simulink model "PD3_DCS_810698349"  (R2021b)
settings: Solver=VariableStepAuto  StartTime=0.0  StopTime=0.1  RelTol=1e-3
undefined symbols (not defined in the file): Ad, C, C_d, G, g, G_d, H, K, Kc, L, L_d, L_p, M, N, R, Ts, wd, y0, y00
settings Model: Creator=SinaK  LastModifiedBy=SinaK

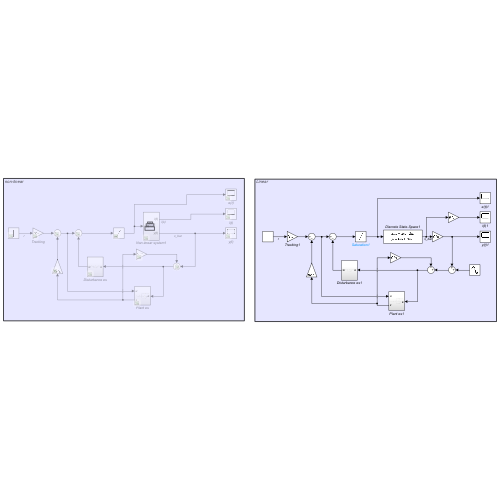
[thumbnail: Simulink's stored preview of the top-level diagram]
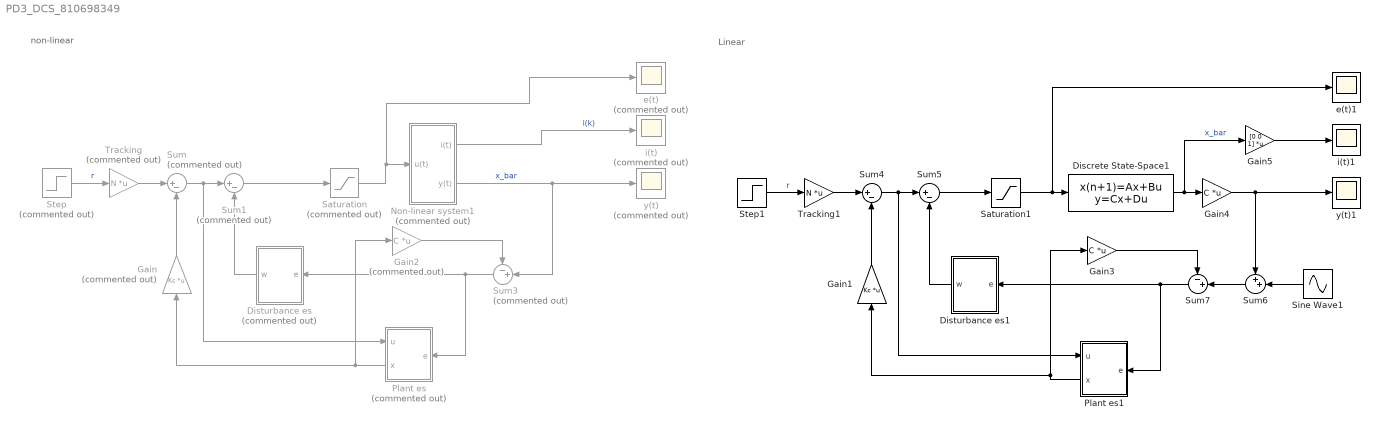
== system PD3_DCS_810698349 ==
  note: Linear
  note: non-linear
  Discrete State-Space1 : DiscreteStateSpace  A=G  B=H  C=eye(3)  D=[0;0;0]  InitialCondition=[y00 0 0]  SampleTime=Ts
  Disturbance es : Subsystem  Commented=on
      settings: PortSchema="{\"entries\":[{\"content\":{\"sides\":[{\"content\":{\"connectorIds\":[\"Out1\"]},\"type\":\"ConnectorPlacement.EquallySpacedRectSide\",\"uuid\":\"7dd2fe88-ba23-450d-b62f-d7570c7d4a9a\"},{\"content\":{\"connectorIds\":[\"In1\"],\"side\":\"RIGHT\"},\"type\":\"ConnectorPlacement.EquallySpacedRectSide\",\"uuid\":\"0a4220da-270b-4baa-869a-0910f399fc2e\"},{\"content\":{\"connectorIds\":[],\"side\":\"TOP\"},\"type\":\"ConnectorPlacement.EquallySpacedRectSide\",\"uuid\":\"bb1cd4e3-8afb-4066-b34f-6b8e4218f629\"}]},\"type\":\"ConnectorPlacement.EquallySpacedConnector\",\"uuid\":\"247f8fe5-253d-4e7a-bc0a-d05e429903fb\"}],\"packageUris\":[\"http://schema.mathworks.com/mf0/Connector/R2020b\"],\"version\":\"1.0\"}"
  Disturbance es1 : Subsystem
      settings: PortSchema="{\"entries\":[{\"content\":{\"sides\":[{\"content\":{\"connectorIds\":[\"Out1\"]},\"type\":\"ConnectorPlacement.EquallySpacedRectSide\",\"uuid\":\"7dd2fe88-ba23-450d-b62f-d7570c7d4a9a\"},{\"content\":{\"connectorIds\":[\"In1\"],\"side\":\"RIGHT\"},\"type\":\"ConnectorPlacement.EquallySpacedRectSide\",\"uuid\":\"0a4220da-270b-4baa-869a-0910f399fc2e\"},{\"content\":{\"connectorIds\":[],\"side\":\"TOP\"},\"type\":\"ConnectorPlacement.EquallySpacedRectSide\",\"uuid\":\"bb1cd4e3-8afb-4066-b34f-6b8e4218f629\"}]},\"type\":\"ConnectorPlacement.EquallySpacedConnector\",\"uuid\":\"247f8fe5-253d-4e7a-bc0a-d05e429903fb\"}],\"packageUris\":[\"http://schema.mathworks.com/mf0/Connector/R2020b\"],\"version\":\"1.0\"}"
  Gain : Gain  Commented=on  Gain=Kc  Multiplication=Matrix(K*u)
  Gain1 : Gain  Gain=Kc  Multiplication=Matrix(K*u)
  Gain2 : Gain  Commented=on  Gain=C  Multiplication=Matrix(K*u)
  Gain3 : Gain  Gain=C  Multiplication=Matrix(K*u)
  Gain4 : Gain  Gain=C  Multiplication=Matrix(K*u)
  Gain5 : Gain  Gain=[0 0 1]  Multiplication=Matrix(K*u)
  Non-linear system1 : Subsystem  Commented=on
  Plant es : Subsystem  Commented=on
      settings: PortSchema="{\"entries\":[{\"content\":{\"sides\":[{\"content\":{\"connectorIds\":[\"In1\",\"Out1\"]},\"type\":\"ConnectorPlacement.EquallySpacedRectSide\",\"uuid\":\"314f560e-5b7f-4e5c-b02d-8249f7ba5ae3\"},{\"content\":{\"connectorIds\":[\"In2\"],\"side\":\"RIGHT\"},\"type\":\"ConnectorPlacement.EquallySpacedRectSide\",\"uuid\":\"7b9ed6a2-80f4-4af4-bb8e-da5172d833a4\"},{\"content\":{\"connectorIds\":[],\"side\":\"TOP\"},\"type\":\"ConnectorPlacement.EquallySpacedRectSide\",\"uuid\":\"b6b0ea98-fd65-4c0a-95e2-ca3e605f4d55\"}]},\"type\":\"ConnectorPlacement.EquallySpacedConnector\",\"uuid\":\"1548adc4-d2fc-42af-9b44-933c6ce86982\"}],\"packageUris\":[\"http://schema.mathworks.com/mf0/Connector/R2020b\"],\"version\":\"1.0\"}"
  Plant es1 : Subsystem
      settings: PortSchema="{\"entries\":[{\"content\":{\"sides\":[{\"content\":{\"connectorIds\":[\"In1\",\"Out1\"]},\"type\":\"ConnectorPlacement.EquallySpacedRectSide\",\"uuid\":\"314f560e-5b7f-4e5c-b02d-8249f7ba5ae3\"},{\"content\":{\"connectorIds\":[\"In2\"],\"side\":\"RIGHT\"},\"type\":\"ConnectorPlacement.EquallySpacedRectSide\",\"uuid\":\"7b9ed6a2-80f4-4af4-bb8e-da5172d833a4\"},{\"content\":{\"connectorIds\":[],\"side\":\"TOP\"},\"type\":\"ConnectorPlacement.EquallySpacedRectSide\",\"uuid\":\"b6b0ea98-fd65-4c0a-95e2-ca3e605f4d55\"}]},\"type\":\"ConnectorPlacement.EquallySpacedConnector\",\"uuid\":\"1548adc4-d2fc-42af-9b44-933c6ce86982\"}],\"packageUris\":[\"http://schema.mathworks.com/mf0/Connector/R2020b\"],\"version\":\"1.0\"}"
  Saturation : Saturate  Commented=on  UpperLimit=12  LowerLimit=0
  Saturation1 : Saturate  UpperLimit=12  LowerLimit=0
  Sine Wave1 : Sin  Amplitude=Ad/M  Frequency=wd  SampleTime=Ts
  Step : Step  Commented=on  Time=0  After=y0  SampleTime=Ts
  Step1 : Step  Time=0  After=y0  SampleTime=Ts
  Sum : Sum  Commented=on  Inputs=|+-
  Sum1 : Sum  Commented=on  Inputs=|+-
  Sum3 : Sum  Commented=on  Inputs=-+|
  Sum4 : Sum  Inputs=|+-
  Sum5 : Sum  Inputs=|+-
  Sum6 : Sum  Inputs=++|
  Sum7 : Sum  Inputs=-+|
  Tracking : Gain  Commented=on  Gain=N  Multiplication=Matrix(K*u)
  Tracking1 : Gain  Gain=N  Multiplication=Matrix(K*u)
  e(t) : Scope  Commented=on
  e(t)1 : Scope
  i(t) : Scope  Commented=on
  i(t)1 : Scope
  y(t) : Scope  Commented=on
  y(t)1 : Scope
  wires:
  Step/1 -> Tracking/1  "r"
  Tracking/1 -> Sum/1
  Sum/1 -> Plant es/1(u), Sum1/1
  Non-linear system1/2(y(t)) -> y(t)/1, Sum3/2  "x_bar"
  Gain/1 -> Sum/2
  Plant es/1(x) -> Gain2/1, Gain/1
  Disturbance es/1(w) -> Sum1/2
  Sum3/1 -> Disturbance es/1(e), Plant es/2(e)
  Gain2/1 -> Sum3/1
  Saturation/1 -> e(t)/1, Non-linear system1/1(u(t))
  Sum1/1 -> Saturation/1
  Non-linear system1/1(i(t)) -> i(t)/1  "i(k)"
  Sum4/1 -> Plant es1/1(u), Sum5/1
  Step1/1 -> Tracking1/1  "r"
  Gain3/1 -> Sum7/1
  Gain1/1 -> Sum4/2
  Tracking1/1 -> Sum4/1
  Sum7/1 -> Disturbance es1/1(e), Plant es1/2(e)
  Plant es1/1(x) -> Gain3/1, Gain1/1
  Disturbance es1/1(w) -> Sum5/2
  Saturation1/1 -> e(t)1/1, Discrete State-Space1/1
  Sum5/1 -> Saturation1/1
  Discrete State-Space1/1 -> Gain5/1, Gain4/1  "x_bar"
  Gain4/1 -> Sum6/1, y(t)1/1
  Gain5/1 -> i(t)1/1
  Sum6/1 -> Sum7/2
  Sine Wave1/1 -> Sum6/2

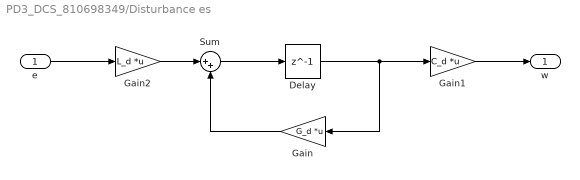
== system PD3_DCS_810698349/Disturbance es ==
  e : Inport
  Delay : Delay  DelayLength=1  SampleTime=Ts
  Gain : Gain  Gain=G_d  Multiplication=Matrix(K*u)
  Gain1 : Gain  Gain=C_d  Multiplication=Matrix(K*u)
  Gain2 : Gain  Gain=L_d  Multiplication=Matrix(K*u)
  Sum : Sum  Inputs=|++
  w : Outport
  wires:
  Sum/1 -> Delay/1
  Gain/1 -> Sum/2
  Delay/1 -> Gain1/1, Gain/1
  Gain1/1 -> w/1
  Gain2/1 -> Sum/1
  e/1 -> Gain2/1

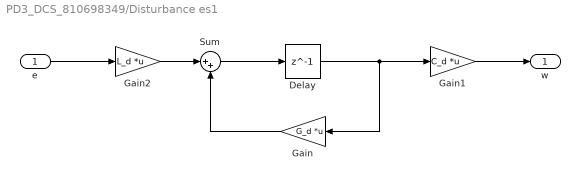
== system PD3_DCS_810698349/Disturbance es1 ==
  e : Inport
  Delay : Delay  DelayLength=1  SampleTime=Ts
  Gain : Gain  Gain=G_d  Multiplication=Matrix(K*u)
  Gain1 : Gain  Gain=C_d  Multiplication=Matrix(K*u)
  Gain2 : Gain  Gain=L_d  Multiplication=Matrix(K*u)
  Sum : Sum  Inputs=|++
  w : Outport
  wires:
  Sum/1 -> Delay/1
  Gain/1 -> Sum/2
  Delay/1 -> Gain1/1, Gain/1
  Gain1/1 -> w/1
  Gain2/1 -> Sum/1
  e/1 -> Gain2/1

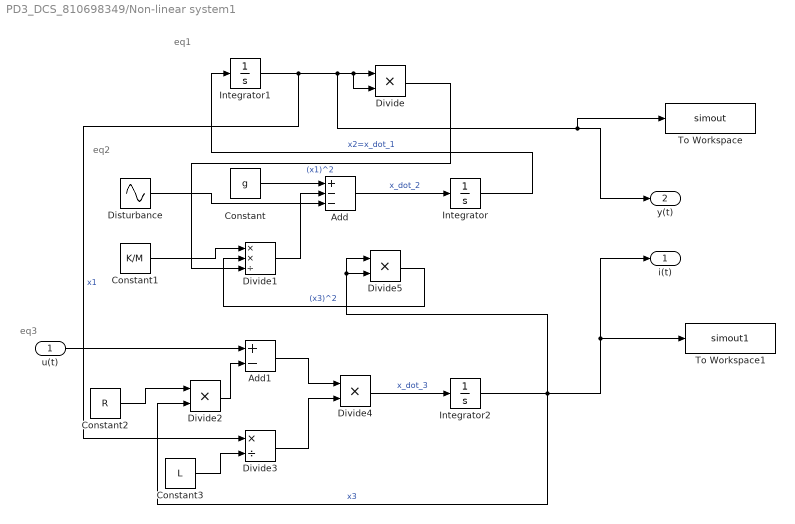
== system PD3_DCS_810698349/Non-linear system1 ==
  note: eq1
  note: eq2
  note: eq3
  u(t) : Inport
  Add : Sum  Inputs=+--
  Add1 : Sum  Inputs=+-
  Constant : Constant  Value=g  SampleTime=Ts
  Constant1 : Constant  Value=K/M  SampleTime=Ts
  Constant2 : Constant  Value=R  SampleTime=Ts
  Constant3 : Constant  Value=L  SampleTime=Ts
  Disturbance : Sin  Amplitude=Ad/M  Frequency=wd  SampleTime=Ts
  Divide{,2,4..5} (4 alike) : Product  Inputs=**
  Divide1 : Product  Inputs=**/
  Divide3 : Product  Inputs=*/
  Integrator : Integrator
  Integrator1 : Integrator  InitialCondition=y00
  Integrator2 : Integrator
  To Workspace : ToWorkspace  VariableName=simout  SaveFormat=Timeseries  SampleTime=-1
      settings: Decimation=3
  To Workspace1 : ToWorkspace  VariableName=simout1  SaveFormat=Timeseries  SampleTime=-1
      settings: Decimation=3
  i(t) : Outport
  y(t) : Outport  Port=2
  wires:
  Add/1 -> Integrator/1  "x_dot_2"
  Divide/1 -> Divide1/3  "(x1)^2"
  Integrator/1 -> Integrator1/1  "x2=x_dot_1"
  Integrator2/1 -> i(t)/1, To Workspace1/1, Divide5/1, Divide5/2, Divide2/2  "x3"
  Divide1/1 -> Add/2
  Add1/1 -> Divide4/1
  Constant3/1 -> Divide3/2
  Constant2/1 -> Divide2/1
  Divide5/1 -> Divide1/2  "(x3)^2"
  Integrator1/1 -> Divide3/1, To Workspace/1, y(t)/1, Divide/2, Divide/1  "x1"
  Divide4/1 -> Integrator2/1  "x_dot_3"
  Constant1/1 -> Divide1/1
  Constant/1 -> Add/1
  Divide3/1 -> Divide4/2
  Divide2/1 -> Add1/2
  u(t)/1 -> Add1/1
  Disturbance/1 -> Add/3

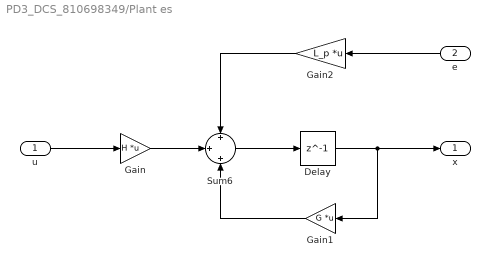
== system PD3_DCS_810698349/Plant es ==
  u : Inport
  e : Inport  Port=2
  Delay : Delay  DelayLength=1  SampleTime=Ts
  Gain : Gain  Gain=H  Multiplication=Matrix(K*u)
  Gain1 : Gain  Gain=G  Multiplication=Matrix(K*u)
  Gain2 : Gain  Gain=L_p  Multiplication=Matrix(K*u)
  Sum6 : Sum  Inputs=+|+|+
  x : Outport
  wires:
  Gain/1 -> Sum6/2
  Sum6/1 -> Delay/1
  Gain1/1 -> Sum6/3
  Delay/1 -> x/1, Gain1/1
  Gain2/1 -> Sum6/1
  e/1 -> Gain2/1
  u/1 -> Gain/1

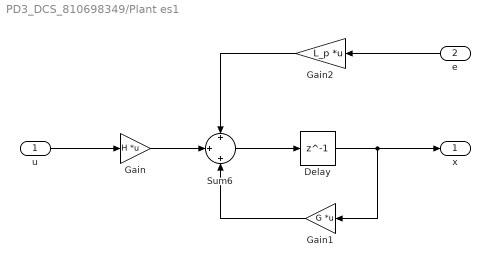
== system PD3_DCS_810698349/Plant es1 ==
  u : Inport
  e : Inport  Port=2
  Delay : Delay  DelayLength=1  SampleTime=Ts
  Gain : Gain  Gain=H  Multiplication=Matrix(K*u)
  Gain1 : Gain  Gain=G  Multiplication=Matrix(K*u)
  Gain2 : Gain  Gain=L_p  Multiplication=Matrix(K*u)
  Sum6 : Sum  Inputs=+|+|+
  x : Outport
  wires:
  Gain/1 -> Sum6/2
  Sum6/1 -> Delay/1
  Gain1/1 -> Sum6/3
  Delay/1 -> x/1, Gain1/1
  Gain2/1 -> Sum6/1
  e/1 -> Gain2/1
  u/1 -> Gain/1
